simulink model "ex_hb1ode"  (R2017a)
settings: Solver=ode15s  StartTime=0.0  StopTime=4e5  FixedStep=0.001  RelTol=1e-3  EnableMultiTasking=on
settings Model: Creator=The MathWorks, Inc.  LastModifiedBy=Vera
settings DataIOCC: LimitDataPoints=on  SaveFormat=Array
settings OptimizationCC: LifeSpan=inf
settings DebuggingCC: SFUnexpectedBacktrackingDiag=warning  SFNoUnconditionalDefaultTransitionDiag=warning  SFExecutionAtInitializationDiag=none
settings HardwareCC: ProdBitPerPointer=32  ProdBitPerSizeT=32  ProdBitPerPtrDiffT=32  ProdLargestAtomicFloat=None  ProdIntDivRoundTo=Undefined  ProdEndianess=Unspecified  ProdWordSize=32  ProdHWDeviceType=32-bit Generic
settings ModelReferenceCC: PropagateSignalLabelsOutOfModel=off
settings GRTTargetCC: TargetLangStandard=C89/C90 (ANSI)  GeneratePreprocessorConditionals=Disable all
settings ConfigComp: CovMetricSettings=dw  CovHtmlReporting=on  CovSaveCumulativeToWorkspaceVar=on  CovSaveSingleToWorkspaceVar=on  CovExternalEMLEnable=off  CovSFcnEnable=off

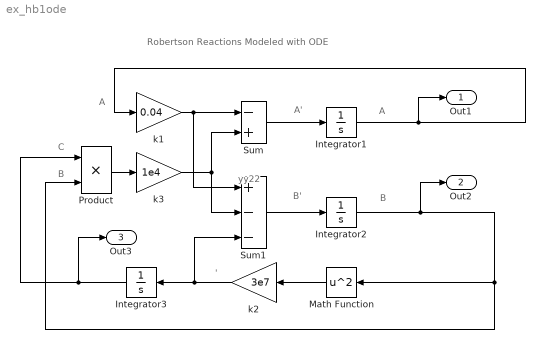
== system ex_hb1ode ==
  note: Robertson Reactions Modeled with ODE
  note: A
  note: B'
  note: A'
  note: B
  note: C
  note: B
  note: A
  note: '
  note: yy22
  Integrator1 : Integrator  InitialCondition=1
  Integrator2 : Integrator
  Integrator3 : Integrator
  Math Function : Math  Operator=square  SaturateOnIntegerOverflow=on
  Product : Product
  Sum : Sum  Inputs=-+
  Sum1 : Sum  Inputs=+--
  k1 : Gain  Gain=0.04
  k2 : Gain  Gain=3e7
  k3 : Gain  Gain=1e4
  Out1 : Outport
  Out2 : Outport  Port=2
  Out3 : Outport  Port=3
  wires:
  Math Function/1 -> k2/1
  k2/1 -> Sum1/3, Integrator3/1
  Product/1 -> k3/1
  k3/1 -> Sum1/2, Sum/2
  k1/1 -> Sum1/1, Sum/1
  Sum1/1 -> Integrator2/1
  Sum/1 -> Integrator1/1
  Integrator2/1 -> Out2/1, Math Function/1, Product/2
  Integrator1/1 -> Out1/1, k1/1
  Integrator3/1 -> Out3/1, Product/1
